simulink model "dft_8_point"  (R2016b)
settings: Solver=VariableStepDiscrete  StartTime=0.0  StopTime=12/fs  RelTol=1e-3  EnableMultiTasking=on
PreLoadFcn:
  | t = 2;
  | b = 14;
  | 
  | fs = 1;
StartFcn:
  | close all;
StopFcn:
  | % create matrices of Re and Im parts over time - inputs
  | xin_re = [xin_0_re xin_1_re xin_2_re xin_3_re xin_4_re xin_5_re xin_6_re xin_7_re];
  | xin_im = [xin_0_im xin_0_im xin_0_im xin_0_im xin_0_im xin_0_im xin_0_im xin_0_im];
  | 
  | % create matrices of Re and Im parts over time - outputs
  | X_re = [X0_re X1_re X2_re X3_re X4_re X5_re X6_re X7_re];
  | X_im = [X0_im X1_im X2_im X3_im X4_im X5_im X6_im X7_im];
  | 
  | % create vectors of Magnitudes and Angles over time
  | X_mag = [X0_mag X1_mag X2_mag X3_mag X4_mag X5_mag X6_mag X7_mag];
  | X_ang = [X0_ang X1_ang X2_ang X3_ang X4_ang X5_ang X6_ang X7_ang];
  | 
  | 
  | figure(1)
  | hold off
  | plot([0:1:7],xin_re(end,:),'r-o','MarkerFaceColor','r');
  | hold on
  | plot([0:1:7],xin_im(end,:),'b-o','MarkerFaceColor','b');
  | xlabel('Samples');
  | ylabel('Magnitude');
  | title('Input to DFT');
  | legend('Real','Imaginary','Location','EastOutside')
  | grid on;
  | 
  | set(1,'Name','Input to DFT','NumberTitle','off');
  | % setStandardFigSize(1);
  | 
  | figure(2)
  | hold off
  | plot([0:1:7],X_mag(end,:),'k-o','MarkerFaceColor','b');
  | hold on
  | xlabel('Frequency Bin');
  | ylabel('Magnitude');
  | grid on;
  | title('Magnitude DFT Plot');
  | 
  | set(2,'Name','Output of DFT','NumberTitle','off');
  | % setStandardFigSize(2);
libraries: xbsIndex_r4 x955
(part 1 of 8)
settings Model: Creator=lcrockett  LastModifiedBy=Administrator
settings DataIOCC: LimitDataPoints=on  SaveFormat=Array  SignalLoggingSaveFormat=ModelDataLogs
settings OptimizationCC: ExpressionDepthLimit=2147483647  LifeSpan=inf
settings DebuggingCC: UnderspecifiedInitializationDetection=Classic  MergeDetectMultiDrivingBlocksExec=none  SolverPrmCheckMsg=warning  FcnCallInpInsideContextMsg=warning  StateNameClashWarn=warning  SFUnexpectedBacktrackingDiag=warning  SFNoUnconditionalDefaultTransitionDiag=warning  SFExecutionAtInitializationDiag=none
settings HardwareCC: ProdBitPerPointer=32  ProdBitPerSizeT=32  ProdBitPerPtrDiffT=32  ProdLargestAtomicFloat=None  ProdIntDivRoundTo=Undefined  ProdEndianess=Unspecified  ProdWordSize=32  ProdHWDeviceType=32-bit Generic
settings ModelReferenceCC: PropagateSignalLabelsOutOfModel=off
settings GRTTargetCC: TargetLangStandard=C89/C90 (ANSI)  GeneratePreprocessorConditionals=Disable all  CombineOutputUpdateFcns=off  GRTInterface=on
settings ConfigComp: CovMetricSettings=dw  CovHtmlReporting=on  CovSaveCumulativeToWorkspaceVar=on  CovSaveSingleToWorkspaceVar=on  CovExternalEMLEnable=off

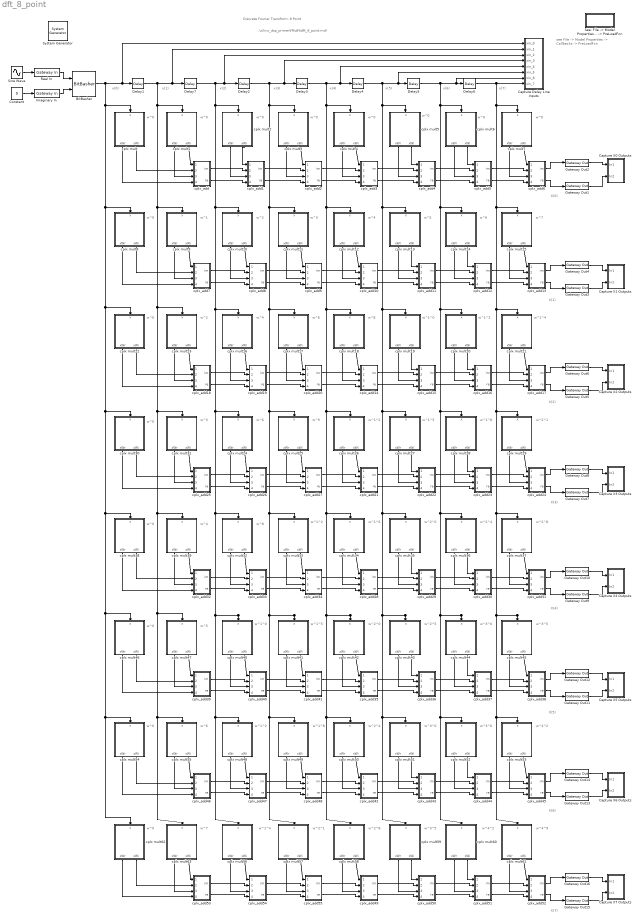
== system dft_8_point ==
  note: w^0
  note: w^0
  note: w^0
  note: w^0
  note: w^0
  note: w^0
  note: w^0
  note: w^0
  note: w^0
  note: w^0
  note: w^0
  note: w^0
  note: w^0
  note: w^0
  note: w^0
  note: w^1
  note: w^2
  note: w^2
  note: w^3
  note: w^3
  note: w^4
  note: w^4
  note: w^5
  note: w^6
  note: w^7
  note: w^5
  note: w^6
  note: w^7
  note: w^4
  note: w^6
  note: w^8
  note: w^1^0
  note: w^1^2
  note: w^1^4
  note: w^6
  note: w^9
  note: w^1^2
  note: w^1^5
  note: w^1^8
  note: w^2^1
  note: w^8
  note: w^1^2
  note: w^1^6
  note: w^2^0
  note: w^2^4
  note: w^2^8
  note: w^1^0
  note: w^1^5
  note: w^2^0
  note: w^2^5
  note: w^3^0
  note: w^3^5
  note: w^1^2
  note: w^1^8
  note: w^2^4
  note: w^3^0
  note: w^3^6
  note: w^4^2
  note: w^1^4
  note: w^2^1
  note: w^2^8
  note: w^3^5
  note: w^4^2
  note: w^4^9
  note: Discrete Fourier Transform: 8 Point
  note: ..\xilinx_dsp_primer\fft\dft\dft_8_point.mdl
  note: see File -> Model Properties
      | -> Callbacks -> PreLoadFcn
  note: x(0)
  note: x(1)
  note: x(2)
  note: x(3)
  note: x(4)
  note: x(5)
  note: x(6)
  note: x(7)
  note: X(0)
  note: X(1)
  note: X(2)
  note: X(3)
  note: X(4)
  note: X(5)
  note: X(6)
  note: X(7)
  " System Generator" : xbsIndex_r4/ System Generator  Tag=genX  xilinxfamily=artix7  part=xc7a75t  speed=-1  package=fgg484  synthesis_tool=Vivado  clock_wrapper=Clock Enables  directory=./netlist  proj_type=Vivado  Synth_file=Vivado Synthesis Defaults  Impl_file=Vivado Implementation Defaults  testbench=off  simulink_period=1/fs  sysclk_period=10  dcm_input_clock_period=10  incr_netlist=off  trim_vbits=Everywhere in SubSystem  dbl_ovrd=According to Block Masks  core_generation=According to Block Masks  run_coregen=off  deprecated_control=off  eval_field=0  block_type=sysgen
  BitBasher : xbsIndex_r4/BitBasher  bitexpr=|  display_expr=on  sr_1=1  arith_type1=Unsigned  bin_pt1=0  sr_2=2  arith_type2=Unsigned  bin_pt2=0  sr_3=3  arith_type3=Unsigned  bin_pt3=0  sr_4=4  arith_type4=Unsigned  bin_pt4=0  dbl_ovrd=off  block_type=bitbasher
      | <!DOCTYPE HTML PUBLIC "-//W3C//DTD HTML 4.0//EN" "http://www.w3.org/TR/REC-html40/strict.dtd">
      | <html><head><meta name="qrichtext" content="1" /><style type="text/css">
      | p, li { white-space: pre-wrap; }
      | </style></head><body style=" font-family:'MS Shell Dlg 2'; font-size:8.25pt; font-weight:400; font-style:normal;">
      | <p style=" margin-top:12px; margin-bottom:12px; margin-left:0px; margin-right:0px; -qt-block-indent:0; text-indent:0px;"><span style=" font-family:'MS Shell Dlg'; font-size:8pt;">a={b,c}</span></p></body></html>
  Capture X0 Outputs : Subsystem
  Capture X2 Outputs : Subsystem
  Capture X6 Outputs : Subsystem
  Capture X1 Outputs : Subsystem
  Capture X3 Outputs : Subsystem
  Capture X4 Outputs : Subsystem
  Capture X5 Outputs : Subsystem
  Capture X7 Outputs : Subsystem
  Capture Delay Line Inputs : Subsystem
  Constant : Constant  Value=0
  Delay{1..7} (7 alike) : xbsIndex_r4/Delay  rst=off  infoeditControl=Selection of Reset will increase slice count due to use of real FFs and instead of SRLs  en=off  latency=1  reg_retiming=off  dbl_ovrd=off  block_type=delay
  Gateway Out{1..16} (16 alike) : xbsIndex_r4/Gateway Out  inherit_from_input=off  hdl_port=on  rows=1  columns=1  UseAsDAC=off  DACChannel='1'  interface=None  automatic_assignment=on  address_offset=hex2dec('00')  intf_name=''  intf_description=''  timing_constraint=None  locs_specified=off  LOCs={}  io_standard={}  block_type=gatewayout
      settings: infoedit="Gateway out block.  Converts Xilinx fixed point inputs into ouputs of type Simulink integer, double, or fixed point.<br><br>Hardware notes:  In hardware these blocks become top level output ports or are discarded, depending on how they are configured."
  Imaginary In : xbsIndex_r4/Gateway In  gui_display_data_type=Fixed-point  arith_type="Signed  (2's comp)"  n_bits=t+b  bin_pt=b  preci_type=Single  exp_width=8  frac_width=24  rows=1  columns=1  quantization="Round  (unbiased: +/- Inf)"  overflow=Saturate  period=1/fs  UseAsADC=off  ADCChannel='1'  interface=None  automatic_assignment=on  address_offset=hex2dec('00')  intf_name=''  intf_description=''  default_value=0  timing_constraint=None  locs_specified=off  LOCs={}  io_standard={}  inherit_from_input=off  hdl_port=on  dbl_ovrd=off  block_type=gatewayin
      settings: infoedit="Gateway in block.  Converts inputs of type Simulink integer, double and fixed point to  Xilinx fixed point type.<br><br>Hardware notes:  In hardware these blocks become top level input ports."
  Real In : xbsIndex_r4/Gateway In  gui_display_data_type=Fixed-point  arith_type="Signed  (2's comp)"  n_bits=t+b  bin_pt=b  preci_type=Single  exp_width=8  frac_width=24  rows=1  columns=1  quantization="Round  (unbiased: +/- Inf)"  overflow=Saturate  period=1/fs  UseAsADC=off  ADCChannel='1'  interface=None  automatic_assignment=on  address_offset=hex2dec('00')  intf_name=''  intf_description=''  default_value=0  timing_constraint=None  locs_specified=off  LOCs={}  io_standard={}  inherit_from_input=off  hdl_port=on  dbl_ovrd=off  block_type=gatewayin
      settings: infoedit="Gateway in block.  Converts inputs of type Simulink integer, double and fixed point to  Xilinx fixed point type.<br><br>Hardware notes:  In hardware these blocks become top level input ports."
  "See: File -> Model Properties -> Callbacks -> PreLoadFcn " : Subsystem
      mask Display:
      | MHz = evalin('base', 'MHz');
      | fprintf(['fs = ',num2str(MHz),' MHz']);
  Sine Wave : Sin  Frequency=fs*2*pi/8  SampleTime=0
  cplx mult : Subsystem  mask(Complex Multiplier for DFT){n=0, k=0}
      mask prompts: n "Signal sample index, n"; k "Frequency index, k"
      mask help: This subsystem will multiply a complex input signal, x, with a complex weight value for the DFT/FFT, as defined via the mask.
      mask init:
      | t = evalin('base','t');   % integer bits
      | b = evalin('base','b');   % fractional bits   
      | N = 8;                    % size of FFT
      | W = exp(-1j*2*pi/N);      % the constant W
      | Wnk = W^(n*k);            % the complex twiddle factor for n,k
      | %W_nk_re = real(Wnk);
      | %W_nk_im = imag(Wnk);
      mask Display:
      | %plot([0.5 0.5+(real(Wnk)/0.5)],[0.5 0.5+(imag(Wnk)/0.5)]);
      | fprintf('Re = %+0.3f\r\nIm = %+0.3f',  real(Wnk), imag(Wnk));
  cplx mult1 : Subsystem  mask(Complex Multiplier for DFT){n=1, k=0}
      mask prompts: n "Signal sample index, n"; k "Frequency index, k"
      mask help: This subsystem will multiply a complex input signal, x, with a complex weight value for the DFT/FFT, as defined via the mask.
      mask init: same as dft_8_point/cplx mult
      mask Display:
      | %plot([0.5 0.5+(real(Wnk)/0.5)],[0.5 0.5+(imag(Wnk)/0.5)]);
      | fprintf('Re = %+0.3f\r\nIm = %+0.3f',  real(Wnk), imag(Wnk));
  cplx mult10 : Subsystem  mask(Complex Multiplier for DFT){n=2, k=1}
      mask prompts: n "Signal sample index, n"; k "Frequency index, k"
      mask help: This subsystem will multiply a complex input signal, x, with a complex weight value for the DFT/FFT, as defined via the mask.
      mask init: same as dft_8_point/cplx mult
      mask Display:
      | %plot([0.5 0.5+(real(Wnk)/0.5)],[0.5 0.5+(imag(Wnk)/0.5)]);
      | fprintf('Re = %+0.3f\r\nIm = %+0.3f',  real(Wnk), imag(Wnk));
  cplx mult11 : Subsystem  mask(Complex Multiplier for DFT){n=3, k=1}
      mask prompts: n "Signal sample index, n"; k "Frequency index, k"
      mask help: This subsystem will multiply a complex input signal, x, with a complex weight value for the DFT/FFT, as defined via the mask.
      mask init: same as dft_8_point/cplx mult
      mask Display:
      | %plot([0.5 0.5+(real(Wnk)/0.5)],[0.5 0.5+(imag(Wnk)/0.5)]);
      | fprintf('Re = %+0.3f\r\nIm = %+0.3f',  real(Wnk), imag(Wnk));
  cplx mult12 : Subsystem  mask(Complex Multiplier for DFT){n=4, k=1}
      mask prompts: n "Signal sample index, n"; k "Frequency index, k"
      mask help: This subsystem will multiply a complex input signal, x, with a complex weight value for the DFT/FFT, as defined via the mask.
      mask init: same as dft_8_point/cplx mult
      mask Display:
      | %plot([0.5 0.5+(real(Wnk)/0.5)],[0.5 0.5+(imag(Wnk)/0.5)]);
      | fprintf('Re = %+0.3f\r\nIm = %+0.3f',  real(Wnk), imag(Wnk));
  cplx mult13 : Subsystem  mask(Complex Multiplier for DFT){n=5, k=1}
      mask prompts: n "Signal sample index, n"; k "Frequency index, k"
      mask help: This subsystem will multiply a complex input signal, x, with a complex weight value for the DFT/FFT, as defined via the mask.
      mask init: same as dft_8_point/cplx mult
      mask Display:
      | %plot([0.5 0.5+(real(Wnk)/0.5)],[0.5 0.5+(imag(Wnk)/0.5)]);
      | fprintf('Re = %+0.3f\r\nIm = %+0.3f',  real(Wnk), imag(Wnk));
  cplx mult14 : Subsystem  mask(Complex Multiplier for DFT){n=6, k=1}
      mask prompts: n "Signal sample index, n"; k "Frequency index, k"
      mask help: This subsystem will multiply a complex input signal, x, with a complex weight value for the DFT/FFT, as defined via the mask.
      mask init: same as dft_8_point/cplx mult
      mask Display:
      | %plot([0.5 0.5+(real(Wnk)/0.5)],[0.5 0.5+(imag(Wnk)/0.5)]);
      | fprintf('Re = %+0.3f\r\nIm = %+0.3f',  real(Wnk), imag(Wnk));
  cplx mult15 : Subsystem  mask(Complex Multiplier for DFT){n=7, k=1}
      mask prompts: n "Signal sample index, n"; k "Frequency index, k"
      mask help: This subsystem will multiply a complex input signal, x, with a complex weight value for the DFT/FFT, as defined via the mask.
      mask init: same as dft_8_point/cplx mult
      mask Display:
      | %plot([0.5 0.5+(real(Wnk)/0.5)],[0.5 0.5+(imag(Wnk)/0.5)]);
      | fprintf('Re = %+0.3f\r\nIm = %+0.3f',  real(Wnk), imag(Wnk));
  cplx mult16 : Subsystem  mask(Complex Multiplier for DFT){n=2, k=2}
      mask prompts: n "Signal sample index, n"; k "Frequency index, k"
      mask help: This subsystem will multiply a complex input signal, x, with a complex weight value for the DFT/FFT, as defined via the mask.
      mask init: same as dft_8_point/cplx mult
      mask Display:
      | %plot([0.5 0.5+(real(Wnk)/0.5)],[0.5 0.5+(imag(Wnk)/0.5)]);
      | fprintf('Re = %+0.3f\r\nIm = %+0.3f',  real(Wnk), imag(Wnk));
  cplx mult17 : Subsystem  mask(Complex Multiplier for DFT){n=3, k=2}
      mask prompts: n "Signal sample index, n"; k "Frequency index, k"
      mask help: This subsystem will multiply a complex input signal, x, with a complex weight value for the DFT/FFT, as defined via the mask.
      mask init: same as dft_8_point/cplx mult
      mask Display:
      | %plot([0.5 0.5+(real(Wnk)/0.5)],[0.5 0.5+(imag(Wnk)/0.5)]);
      | fprintf('Re = %+0.3f\r\nIm = %+0.3f',  real(Wnk), imag(Wnk));
  cplx mult18 : Subsystem  mask(Complex Multiplier for DFT){n=4, k=2}
      mask prompts: n "Signal sample index, n"; k "Frequency index, k"
      mask help: This subsystem will multiply a complex input signal, x, with a complex weight value for the DFT/FFT, as defined via the mask.
      mask init: same as dft_8_point/cplx mult
      mask Display:
      | %plot([0.5 0.5+(real(Wnk)/0.5)],[0.5 0.5+(imag(Wnk)/0.5)]);
      | fprintf('Re = %+0.3f\r\nIm = %+0.3f',  real(Wnk), imag(Wnk));
  cplx mult19 : Subsystem  mask(Complex Multiplier for DFT){n=5, k=2}
      mask prompts: n "Signal sample index, n"; k "Frequency index, k"
      mask help: This subsystem will multiply a complex input signal, x, with a complex weight value for the DFT/FFT, as defined via the mask.
      mask init: same as dft_8_point/cplx mult
      mask Display:
      | %plot([0.5 0.5+(real(Wnk)/0.5)],[0.5 0.5+(imag(Wnk)/0.5)]);
      | fprintf('Re = %+0.3f\r\nIm = %+0.3f',  real(Wnk), imag(Wnk));
  cplx mult2 : Subsystem  mask(Complex Multiplier for DFT){n=2, k=0}
      mask prompts: n "Signal sample index, n"; k "Frequency index, k"
      mask help: This subsystem will multiply a complex input signal, x, with a complex weight value for the DFT/FFT, as defined via the mask.
      mask init: same as dft_8_point/cplx mult
      mask Display:
      | %plot([0.5 0.5+(real(Wnk)/0.5)],[0.5 0.5+(imag(Wnk)/0.5)]);
      | fprintf('Re = %+0.3f\r\nIm = %+0.3f',  real(Wnk), imag(Wnk));
  cplx mult20 : Subsystem  mask(Complex Multiplier for DFT){n=6, k=2}
      mask prompts: n "Signal sample index, n"; k "Frequency index, k"
      mask help: This subsystem will multiply a complex input signal, x, with a complex weight value for the DFT/FFT, as defined via the mask.
      mask init: same as dft_8_point/cplx mult
      mask Display:
      | %plot([0.5 0.5+(real(Wnk)/0.5)],[0.5 0.5+(imag(Wnk)/0.5)]);
      | fprintf('Re = %+0.3f\r\nIm = %+0.3f',  real(Wnk), imag(Wnk));
  cplx mult21 : Subsystem  mask(Complex Multiplier for DFT){n=7, k=2}
      mask prompts: n "Signal sample index, n"; k "Frequency index, k"
      mask help: This subsystem will multiply a complex input signal, x, with a complex weight value for the DFT/FFT, as defined via the mask.
      mask init: same as dft_8_point/cplx mult
      mask Display:
      | %plot([0.5 0.5+(real(Wnk)/0.5)],[0.5 0.5+(imag(Wnk)/0.5)]);
      | fprintf('Re = %+0.3f\r\nIm = %+0.3f',  real(Wnk), imag(Wnk));
  cplx mult22 : Subsystem  mask(Complex Multiplier for DFT){n=0, k=2}
      mask prompts: n "Signal sample index, n"; k "Frequency index, k"
      mask help: This subsystem will multiply a complex input signal, x, with a complex weight value for the DFT/FFT, as defined via the mask.
      mask init: same as dft_8_point/cplx mult
      mask Display:
      | %plot([0.5 0.5+(real(Wnk)/0.5)],[0.5 0.5+(imag(Wnk)/0.5)]);
      | fprintf('Re = %+0.3f\r\nIm = %+0.3f',  real(Wnk), imag(Wnk));
  cplx mult23 : Subsystem  mask(Complex Multiplier for DFT){n=1, k=2}
      mask prompts: n "Signal sample index, n"; k "Frequency index, k"
      mask help: This subsystem will multiply a complex input signal, x, with a complex weight value for the DFT/FFT, as defined via the mask.
      mask init: same as dft_8_point/cplx mult
      mask Display:
      | %plot([0.5 0.5+(real(Wnk)/0.5)],[0.5 0.5+(imag(Wnk)/0.5)]);
      | fprintf('Re = %+0.3f\r\nIm = %+0.3f',  real(Wnk), imag(Wnk));
  cplx mult24 : Subsystem  mask(Complex Multiplier for DFT){n=2, k=3}
      mask prompts: n "Signal sample index, n"; k "Frequency index, k"
      mask help: This subsystem will multiply a complex input signal, x, with a complex weight value for the DFT/FFT, as defined via the mask.
      mask init: same as dft_8_point/cplx mult
      mask Display:
      | %plot([0.5 0.5+(real(Wnk)/0.5)],[0.5 0.5+(imag(Wnk)/0.5)]);
      | fprintf('Re = %+0.3f\r\nIm = %+0.3f',  real(Wnk), imag(Wnk));
  cplx mult25 : Subsystem  mask(Complex Multiplier for DFT){n=3, k=3}
      mask prompts: n "Signal sample index, n"; k "Frequency index, k"
      mask help: This subsystem will multiply a complex input signal, x, with a complex weight value for the DFT/FFT, as defined via the mask.
      mask init: same as dft_8_point/cplx mult
      mask Display:
      | %plot([0.5 0.5+(real(Wnk)/0.5)],[0.5 0.5+(imag(Wnk)/0.5)]);
      | fprintf('Re = %+0.3f\r\nIm = %+0.3f',  real(Wnk), imag(Wnk));
  cplx mult26 : Subsystem  mask(Complex Multiplier for DFT){n=4, k=3}
      mask prompts: n "Signal sample index, n"; k "Frequency index, k"
      mask help: This subsystem will multiply a complex input signal, x, with a complex weight value for the DFT/FFT, as defined via the mask.
      mask init: same as dft_8_point/cplx mult
      mask Display:
      | %plot([0.5 0.5+(real(Wnk)/0.5)],[0.5 0.5+(imag(Wnk)/0.5)]);
      | fprintf('Re = %+0.3f\r\nIm = %+0.3f',  real(Wnk), imag(Wnk));
  cplx mult27 : Subsystem  mask(Complex Multiplier for DFT){n=5, k=3}
      mask prompts: n "Signal sample index, n"; k "Frequency index, k"
      mask help: This subsystem will multiply a complex input signal, x, with a complex weight value for the DFT/FFT, as defined via the mask.
      mask init: same as dft_8_point/cplx mult
      mask Display:
      | %plot([0.5 0.5+(real(Wnk)/0.5)],[0.5 0.5+(imag(Wnk)/0.5)]);
      | fprintf('Re = %+0.3f\r\nIm = %+0.3f',  real(Wnk), imag(Wnk));
  cplx mult28 : Subsystem  mask(Complex Multiplier for DFT){n=6, k=3}
      mask prompts: n "Signal sample index, n"; k "Frequency index, k"
      mask help: This subsystem will multiply a complex input signal, x, with a complex weight value for the DFT/FFT, as defined via the mask.
      mask init: same as dft_8_point/cplx mult
      mask Display:
      | %plot([0.5 0.5+(real(Wnk)/0.5)],[0.5 0.5+(imag(Wnk)/0.5)]);
      | fprintf('Re = %+0.3f\r\nIm = %+0.3f',  real(Wnk), imag(Wnk));
  cplx mult29 : Subsystem  mask(Complex Multiplier for DFT){n=7, k=3}
      mask prompts: n "Signal sample index, n"; k "Frequency index, k"
      mask help: This subsystem will multiply a complex input signal, x, with a complex weight value for the DFT/FFT, as defined via the mask.
      mask init: same as dft_8_point/cplx mult
      mask Display:
      | %plot([0.5 0.5+(real(Wnk)/0.5)],[0.5 0.5+(imag(Wnk)/0.5)]);
      | fprintf('Re = %+0.3f\r\nIm = %+0.3f',  real(Wnk), imag(Wnk));
  cplx mult3 : Subsystem  mask(Complex Multiplier for DFT){n=3, k=0}
      mask prompts: n "Signal sample index, n"; k "Frequency index, k"
      mask help: This subsystem will multiply a complex input signal, x, with a complex weight value for the DFT/FFT, as defined via the mask.
      mask init: same as dft_8_point/cplx mult
      mask Display:
      | %plot([0.5 0.5+(real(Wnk)/0.5)],[0.5 0.5+(imag(Wnk)/0.5)]);
      | fprintf('Re = %+0.3f\r\nIm = %+0.3f',  real(Wnk), imag(Wnk));
  cplx mult30 : Subsystem  mask(Complex Multiplier for DFT){n=0, k=3}
      mask prompts: n "Signal sample index, n"; k "Frequency index, k"
      mask help: This subsystem will multiply a complex input signal, x, with a complex weight value for the DFT/FFT, as defined via the mask.
      mask init: same as dft_8_point/cplx mult
      mask Display:
      | %plot([0.5 0.5+(real(Wnk)/0.5)],[0.5 0.5+(imag(Wnk)/0.5)]);
      | fprintf('Re = %+0.3f\r\nIm = %+0.3f',  real(Wnk), imag(Wnk));
  cplx mult31 : Subsystem  mask(Complex Multiplier for DFT){n=1, k=3}
      mask prompts: n "Signal sample index, n"; k "Frequency index, k"
      mask help: This subsystem will multiply a complex input signal, x, with a complex weight value for the DFT/FFT, as defined via the mask.
      mask init: same as dft_8_point/cplx mult
      mask Display:
      | %plot([0.5 0.5+(real(Wnk)/0.5)],[0.5 0.5+(imag(Wnk)/0.5)]);
      | fprintf('Re = %+0.3f\r\nIm = %+0.3f',  real(Wnk), imag(Wnk));
  cplx mult32 : Subsystem  mask(Complex Multiplier for DFT){n=2, k=4}
      mask prompts: n "Signal sample index, n"; k "Frequency index, k"
      mask help: This subsystem will multiply a complex input signal, x, with a complex weight value for the DFT/FFT, as defined via the mask.
      mask init: same as dft_8_point/cplx mult
      mask Display:
      | %plot([0.5 0.5+(real(Wnk)/0.5)],[0.5 0.5+(imag(Wnk)/0.5)]);
      | fprintf('Re = %+0.3f\r\nIm = %+0.3f',  real(Wnk), imag(Wnk));
  cplx mult33 : Subsystem  mask(Complex Multiplier for DFT){n=3, k=4}
      mask prompts: n "Signal sample index, n"; k "Frequency index, k"
      mask help: This subsystem will multiply a complex input signal, x, with a complex weight value for the DFT/FFT, as defined via the mask.
      mask init: same as dft_8_point/cplx mult
      mask Display:
      | %plot([0.5 0.5+(real(Wnk)/0.5)],[0.5 0.5+(imag(Wnk)/0.5)]);
      | fprintf('Re = %+0.3f\r\nIm = %+0.3f',  real(Wnk), imag(Wnk));
  cplx mult34 : Subsystem  mask(Complex Multiplier for DFT){n=4, k=4}
      mask prompts: n "Signal sample index, n"; k "Frequency index, k"
      mask help: This subsystem will multiply a complex input signal, x, with a complex weight value for the DFT/FFT, as defined via the mask.
      mask init: same as dft_8_point/cplx mult
      mask Display:
      | %plot([0.5 0.5+(real(Wnk)/0.5)],[0.5 0.5+(imag(Wnk)/0.5)]);
      | fprintf('Re = %+0.3f\r\nIm = %+0.3f',  real(Wnk), imag(Wnk));
  cplx mult35 : Subsystem  mask(Complex Multiplier for DFT){n=5, k=4}
      mask prompts: n "Signal sample index, n"; k "Frequency index, k"
      mask help: This subsystem will multiply a complex input signal, x, with a complex weight value for the DFT/FFT, as defined via the mask.
      mask init: same as dft_8_point/cplx mult
      mask Display:
      | %plot([0.5 0.5+(real(Wnk)/0.5)],[0.5 0.5+(imag(Wnk)/0.5)]);
      | fprintf('Re = %+0.3f\r\nIm = %+0.3f',  real(Wnk), imag(Wnk));
  cplx mult36 : Subsystem  mask(Complex Multiplier for DFT){n=6, k=4}
      mask prompts: n "Signal sample index, n"; k "Frequency index, k"
      mask help: This subsystem will multiply a complex input signal, x, with a complex weight value for the DFT/FFT, as defined via the mask.
      mask init: same as dft_8_point/cplx mult
      mask Display:
      | %plot([0.5 0.5+(real(Wnk)/0.5)],[0.5 0.5+(imag(Wnk)/0.5)]);
      | fprintf('Re = %+0.3f\r\nIm = %+0.3f',  real(Wnk), imag(Wnk));
  cplx mult37 : Subsystem  mask(Complex Multiplier for DFT){n=7, k=4}
      mask prompts: n "Signal sample index, n"; k "Frequency index, k"
      mask help: This subsystem will multiply a complex input signal, x, with a complex weight value for the DFT/FFT, as defined via the mask.
      mask init: same as dft_8_point/cplx mult
      mask Display:
      | %plot([0.5 0.5+(real(Wnk)/0.5)],[0.5 0.5+(imag(Wnk)/0.5)]);
      | fprintf('Re = %+0.3f\r\nIm = %+0.3f',  real(Wnk), imag(Wnk));
  cplx mult38 : Subsystem  mask(Complex Multiplier for DFT){n=0, k=4}
      mask prompts: n "Signal sample index, n"; k "Frequency index, k"
      mask help: This subsystem will multiply a complex input signal, x, with a complex weight value for the DFT/FFT, as defined via the mask.
      mask init: same as dft_8_point/cplx mult
      mask Display:
      | %plot([0.5 0.5+(real(Wnk)/0.5)],[0.5 0.5+(imag(Wnk)/0.5)]);
      | fprintf('Re = %+0.3f\r\nIm = %+0.3f',  real(Wnk), imag(Wnk));
  cplx mult39 : Subsystem  mask(Complex Multiplier for DFT){n=1, k=4}
      mask prompts: n "Signal sample index, n"; k "Frequency index, k"
      mask help: This subsystem will multiply a complex input signal, x, with a complex weight value for the DFT/FFT, as defined via the mask.
      mask init: same as dft_8_point/cplx mult
      mask Display:
      | %plot([0.5 0.5+(real(Wnk)/0.5)],[0.5 0.5+(imag(Wnk)/0.5)]);
      | fprintf('Re = %+0.3f\r\nIm = %+0.3f',  real(Wnk), imag(Wnk));
  cplx mult4 : Subsystem  mask(Complex Multiplier for DFT){n=4, k=0}
      mask prompts: n "Signal sample index, n"; k "Frequency index, k"
      mask help: This subsystem will multiply a complex input signal, x, with a complex weight value for the DFT/FFT, as defined via the mask.
      mask init: same as dft_8_point/cplx mult
      mask Display:
      | %plot([0.5 0.5+(real(Wnk)/0.5)],[0.5 0.5+(imag(Wnk)/0.5)]);
      | fprintf('Re = %+0.3f\r\nIm = %+0.3f',  real(Wnk), imag(Wnk));
  cplx mult40 : Subsystem  mask(Complex Multiplier for DFT){n=2, k=5}
      mask prompts: n "Signal sample index, n"; k "Frequency index, k"
      mask help: This subsystem will multiply a complex input signal, x, with a complex weight value for the DFT/FFT, as defined via the mask.
      mask init: same as dft_8_point/cplx mult
      mask Display:
      | %plot([0.5 0.5+(real(Wnk)/0.5)],[0.5 0.5+(imag(Wnk)/0.5)]);
      | fprintf('Re = %+0.3f\r\nIm = %+0.3f',  real(Wnk), imag(Wnk));
  cplx mult41 : Subsystem  mask(Complex Multiplier for DFT){n=3, k=5}
      mask prompts: n "Signal sample index, n"; k "Frequency index, k"
      mask help: This subsystem will multiply a complex input signal, x, with a complex weight value for the DFT/FFT, as defined via the mask.
      mask init: same as dft_8_point/cplx mult
      mask Display:
      | %plot([0.5 0.5+(real(Wnk)/0.5)],[0.5 0.5+(imag(Wnk)/0.5)]);
      | fprintf('Re = %+0.3f\r\nIm = %+0.3f',  real(Wnk), imag(Wnk));
  cplx mult42 : Subsystem  mask(Complex Multiplier for DFT){n=4, k=5}
      mask prompts: n "Signal sample index, n"; k "Frequency index, k"
      mask help: This subsystem will multiply a complex input signal, x, with a complex weight value for the DFT/FFT, as defined via the mask.
      mask init: same as dft_8_point/cplx mult
      mask Display:
      | %plot([0.5 0.5+(real(Wnk)/0.5)],[0.5 0.5+(imag(Wnk)/0.5)]);
      | fprintf('Re = %+0.3f\r\nIm = %+0.3f',  real(Wnk), imag(Wnk));
  cplx mult43 : Subsystem  mask(Complex Multiplier for DFT){n=5, k=5}
      mask prompts: n "Signal sample index, n"; k "Frequency index, k"
      mask help: This subsystem will multiply a complex input signal, x, with a complex weight value for the DFT/FFT, as defined via the mask.
      mask init: same as dft_8_point/cplx mult
      mask Display:
      | %plot([0.5 0.5+(real(Wnk)/0.5)],[0.5 0.5+(imag(Wnk)/0.5)]);
      | fprintf('Re = %+0.3f\r\nIm = %+0.3f',  real(Wnk), imag(Wnk));
  cplx mult44 : Subsystem  mask(Complex Multiplier for DFT){n=6, k=5}
      mask prompts: n "Signal sample index, n"; k "Frequency index, k"
      mask help: This subsystem will multiply a complex input signal, x, with a complex weight value for the DFT/FFT, as defined via the mask.
      mask init: same as dft_8_point/cplx mult
      mask Display:
      | %plot([0.5 0.5+(real(Wnk)/0.5)],[0.5 0.5+(imag(Wnk)/0.5)]);
      | fprintf('Re = %+0.3f\r\nIm = %+0.3f',  real(Wnk), imag(Wnk));
  cplx mult45 : Subsystem  mask(Complex Multiplier for DFT){n=7, k=5}
      mask prompts: n "Signal sample index, n"; k "Frequency index, k"
      mask help: This subsystem will multiply a complex input signal, x, with a complex weight value for the DFT/FFT, as defined via the mask.
      mask init: same as dft_8_point/cplx mult
      mask Display:
      | %plot([0.5 0.5+(real(Wnk)/0.5)],[0.5 0.5+(imag(Wnk)/0.5)]);
      | fprintf('Re = %+0.3f\r\nIm = %+0.3f',  real(Wnk), imag(Wnk));
  cplx mult46 : Subsystem  mask(Complex Multiplier for DFT){n=0, k=5}
      mask prompts: n "Signal sample index, n"; k "Frequency index, k"
      mask help: This subsystem will multiply a complex input signal, x, with a complex weight value for the DFT/FFT, as defined via the mask.
      mask init: same as dft_8_point/cplx mult
      mask Display:
      | %plot([0.5 0.5+(real(Wnk)/0.5)],[0.5 0.5+(imag(Wnk)/0.5)]);
      | fprintf('Re = %+0.3f\r\nIm = %+0.3f',  real(Wnk), imag(Wnk));
  cplx mult47 : Subsystem  mask(Complex Multiplier for DFT){n=1, k=5}
      mask prompts: n "Signal sample index, n"; k "Frequency index, k"
      mask help: This subsystem will multiply a complex input signal, x, with a complex weight value for the DFT/FFT, as defined via the mask.
      mask init: same as dft_8_point/cplx mult
      mask Display:
      | %plot([0.5 0.5+(real(Wnk)/0.5)],[0.5 0.5+(imag(Wnk)/0.5)]);
      | fprintf('Re = %+0.3f\r\nIm = %+0.3f',  real(Wnk), imag(Wnk));
  cplx mult48 : Subsystem  mask(Complex Multiplier for DFT){n=2, k=6}
      mask prompts: n "Signal sample index, n"; k "Frequency index, k"
      mask help: This subsystem will multiply a complex input signal, x, with a complex weight value for the DFT/FFT, as defined via the mask.
      mask init: same as dft_8_point/cplx mult
      mask Display:
      | %plot([0.5 0.5+(real(Wnk)/0.5)],[0.5 0.5+(imag(Wnk)/0.5)]);
      | fprintf('Re = %+0.3f\r\nIm = %+0.3f',  real(Wnk), imag(Wnk));
  cplx mult49 : Subsystem  mask(Complex Multiplier for DFT){n=3, k=6}
      mask prompts: n "Signal sample index, n"; k "Frequency index, k"
      mask help: This subsystem will multiply a complex input signal, x, with a complex weight value for the DFT/FFT, as defined via the mask.
      mask init: same as dft_8_point/cplx mult
      mask Display:
      | %plot([0.5 0.5+(real(Wnk)/0.5)],[0.5 0.5+(imag(Wnk)/0.5)]);
      | fprintf('Re = %+0.3f\r\nIm = %+0.3f',  real(Wnk), imag(Wnk));
  cplx mult5 : Subsystem  mask(Complex Multiplier for DFT){n=5, k=0}
      mask prompts: n "Signal sample index, n"; k "Frequency index, k"
      mask help: This subsystem will multiply a complex input signal, x, with a complex weight value for the DFT/FFT, as defined via the mask.
      mask init: same as dft_8_point/cplx mult
      mask Display:
      | %plot([0.5 0.5+(real(Wnk)/0.5)],[0.5 0.5+(imag(Wnk)/0.5)]);
      | fprintf('Re = %+0.3f\r\nIm = %+0.3f',  real(Wnk), imag(Wnk));
  cplx mult50 : Subsystem  mask(Complex Multiplier for DFT){n=4, k=6}
      mask prompts: n "Signal sample index, n"; k "Frequency index, k"
      mask help: This subsystem will multiply a complex input signal, x, with a complex weight value for the DFT/FFT, as defined via the mask.
      mask init: same as dft_8_point/cplx mult
      mask Display:
      | %plot([0.5 0.5+(real(Wnk)/0.5)],[0.5 0.5+(imag(Wnk)/0.5)]);
      | fprintf('Re = %+0.3f\r\nIm = %+0.3f',  real(Wnk), imag(Wnk));
  cplx mult51 : Subsystem  mask(Complex Multiplier for DFT){n=5, k=6}
      mask prompts: n "Signal sample index, n"; k "Frequency index, k"
      mask help: This subsystem will multiply a complex input signal, x, with a complex weight value for the DFT/FFT, as defined via the mask.
      mask init: same as dft_8_point/cplx mult
      mask Display:
      | %plot([0.5 0.5+(real(Wnk)/0.5)],[0.5 0.5+(imag(Wnk)/0.5)]);
      | fprintf('Re = %+0.3f\r\nIm = %+0.3f',  real(Wnk), imag(Wnk));
  cplx mult52 : Subsystem  mask(Complex Multiplier for DFT){n=6, k=6}
      mask prompts: n "Signal sample index, n"; k "Frequency index, k"
      mask help: This subsystem will multiply a complex input signal, x, with a complex weight value for the DFT/FFT, as defined via the mask.
      mask init: same as dft_8_point/cplx mult
      mask Display:
      | %plot([0.5 0.5+(real(Wnk)/0.5)],[0.5 0.5+(imag(Wnk)/0.5)]);
      | fprintf('Re = %+0.3f\r\nIm = %+0.3f',  real(Wnk), imag(Wnk));
  cplx mult53 : Subsystem  mask(Complex Multiplier for DFT){n=7, k=6}
      mask prompts: n "Signal sample index, n"; k "Frequency index, k"
      mask help: This subsystem will multiply a complex input signal, x, with a complex weight value for the DFT/FFT, as defined via the mask.
      mask init: same as dft_8_point/cplx mult
      mask Display:
      | %plot([0.5 0.5+(real(Wnk)/0.5)],[0.5 0.5+(imag(Wnk)/0.5)]);
      | fprintf('Re = %+0.3f\r\nIm = %+0.3f',  real(Wnk), imag(Wnk));
  cplx mult54 : Subsystem  mask(Complex Multiplier for DFT){n=0, k=6}
      mask prompts: n "Signal sample index, n"; k "Frequency index, k"
      mask help: This subsystem will multiply a complex input signal, x, with a complex weight value for the DFT/FFT, as defined via the mask.
      mask init: same as dft_8_point/cplx mult
      mask Display:
      | %plot([0.5 0.5+(real(Wnk)/0.5)],[0.5 0.5+(imag(Wnk)/0.5)]);
      | fprintf('Re = %+0.3f\r\nIm = %+0.3f',  real(Wnk), imag(Wnk));
  cplx mult55 : Subsystem  mask(Complex Multiplier for DFT){n=1, k=6}
      mask prompts: n "Signal sample index, n"; k "Frequency index, k"
      mask help: This subsystem will multiply a complex input signal, x, with a complex weight value for the DFT/FFT, as defined via the mask.
      mask init: same as dft_8_point/cplx mult
      mask Display:
      | %plot([0.5 0.5+(real(Wnk)/0.5)],[0.5 0.5+(imag(Wnk)/0.5)]);
      | fprintf('Re = %+0.3f\r\nIm = %+0.3f',  real(Wnk), imag(Wnk));
  cplx mult56 : Subsystem  mask(Complex Multiplier for DFT){n=2, k=7}
      mask prompts: n "Signal sample index, n"; k "Frequency index, k"
      mask help: This subsystem will multiply a complex input signal, x, with a complex weight value for the DFT/FFT, as defined via the mask.
      mask init: same as dft_8_point/cplx mult
      mask Display:
      | %plot([0.5 0.5+(real(Wnk)/0.5)],[0.5 0.5+(imag(Wnk)/0.5)]);
      | fprintf('Re = %+0.3f\r\nIm = %+0.3f',  real(Wnk), imag(Wnk));
  cplx mult57 : Subsystem  mask(Complex Multiplier for DFT){n=3, k=7}
      mask prompts: n "Signal sample index, n"; k "Frequency index, k"
      mask help: This subsystem will multiply a complex input signal, x, with a complex weight value for the DFT/FFT, as defined via the mask.
      mask init: same as dft_8_point/cplx mult
      mask Display:
      | %plot([0.5 0.5+(real(Wnk)/0.5)],[0.5 0.5+(imag(Wnk)/0.5)]);
      | fprintf('Re = %+0.3f\r\nIm = %+0.3f',  real(Wnk), imag(Wnk));
  cplx mult58 : Subsystem  mask(Complex Multiplier for DFT){n=4, k=7}
      mask prompts: n "Signal sample index, n"; k "Frequency index, k"
      mask help: This subsystem will multiply a complex input signal, x, with a complex weight value for the DFT/FFT, as defined via the mask.
      mask init: same as dft_8_point/cplx mult
      mask Display:
      | %plot([0.5 0.5+(real(Wnk)/0.5)],[0.5 0.5+(imag(Wnk)/0.5)]);
      | fprintf('Re = %+0.3f\r\nIm = %+0.3f',  real(Wnk), imag(Wnk));
  cplx mult59 : Subsystem  mask(Complex Multiplier for DFT){n=5, k=7}
      mask prompts: n "Signal sample index, n"; k "Frequency index, k"
      mask help: This subsystem will multiply a complex input signal, x, with a complex weight value for the DFT/FFT, as defined via the mask.
      mask init: same as dft_8_point/cplx mult
      mask Display:
      | %plot([0.5 0.5+(real(Wnk)/0.5)],[0.5 0.5+(imag(Wnk)/0.5)]);
      | fprintf('Re = %+0.3f\r\nIm = %+0.3f',  real(Wnk), imag(Wnk));
  cplx mult6 : Subsystem  mask(Complex Multiplier for DFT){n=6, k=0}
      mask prompts: n "Signal sample index, n"; k "Frequency index, k"
      mask help: This subsystem will multiply a complex input signal, x, with a complex weight value for the DFT/FFT, as defined via the mask.
      mask init: same as dft_8_point/cplx mult
      mask Display:
      | %plot([0.5 0.5+(real(Wnk)/0.5)],[0.5 0.5+(imag(Wnk)/0.5)]);
      | fprintf('Re = %+0.3f\r\nIm = %+0.3f',  real(Wnk), imag(Wnk));
  cplx mult60 : Subsystem  mask(Complex Multiplier for DFT){n=6, k=7}
      mask prompts: n "Signal sample index, n"; k "Frequency index, k"
      mask help: This subsystem will multiply a complex input signal, x, with a complex weight value for the DFT/FFT, as defined via the mask.
      mask init: same as dft_8_point/cplx mult
      mask Display:
      | %plot([0.5 0.5+(real(Wnk)/0.5)],[0.5 0.5+(imag(Wnk)/0.5)]);
      | fprintf('Re = %+0.3f\r\nIm = %+0.3f',  real(Wnk), imag(Wnk));
  cplx mult61 : Subsystem  mask(Complex Multiplier for DFT){n=7, k=7}
      mask prompts: n "Signal sample index, n"; k "Frequency index, k"
      mask help: This subsystem will multiply a complex input signal, x, with a complex weight value for the DFT/FFT, as defined via the mask.
      mask init: same as dft_8_point/cplx mult
      mask Display:
      | %plot([0.5 0.5+(real(Wnk)/0.5)],[0.5 0.5+(imag(Wnk)/0.5)]);
      | fprintf('Re = %+0.3f\r\nIm = %+0.3f',  real(Wnk), imag(Wnk));
  cplx mult62 : Subsystem  mask(Complex Multiplier for DFT){n=0, k=7}
      mask prompts: n "Signal sample index, n"; k "Frequency index, k"
      mask help: This subsystem will multiply a complex input signal, x, with a complex weight value for the DFT/FFT, as defined via the mask.
      mask init: same as dft_8_point/cplx mult
      mask Display:
      | %plot([0.5 0.5+(real(Wnk)/0.5)],[0.5 0.5+(imag(Wnk)/0.5)]);
      | fprintf('Re = %+0.3f\r\nIm = %+0.3f',  real(Wnk), imag(Wnk));
  cplx mult63 : Subsystem  mask(Complex Multiplier for DFT){n=1, k=7}
      mask prompts: n "Signal sample index, n"; k "Frequency index, k"
      mask help: This subsystem will multiply a complex input signal, x, with a complex weight value for the DFT/FFT, as defined via the mask.
      mask init: same as dft_8_point/cplx mult
      mask Display:
      | %plot([0.5 0.5+(real(Wnk)/0.5)],[0.5 0.5+(imag(Wnk)/0.5)]);
      | fprintf('Re = %+0.3f\r\nIm = %+0.3f',  real(Wnk), imag(Wnk));
  cplx mult7 : Subsystem  mask(Complex Multiplier for DFT){n=7, k=0}
      mask prompts: n "Signal sample index, n"; k "Frequency index, k"
      mask help: This subsystem will multiply a complex input signal, x, with a complex weight value for the DFT/FFT, as defined via the mask.
      mask init: same as dft_8_point/cplx mult
      mask Display:
      | %plot([0.5 0.5+(real(Wnk)/0.5)],[0.5 0.5+(imag(Wnk)/0.5)]);
      | fprintf('Re = %+0.3f\r\nIm = %+0.3f',  real(Wnk), imag(Wnk));
  cplx mult8 : Subsystem  mask(Complex Multiplier for DFT){n=0, k=1}
      mask prompts: n "Signal sample index, n"; k "Frequency index, k"
      mask help: This subsystem will multiply a complex input signal, x, with a complex weight value for the DFT/FFT, as defined via the mask.
      mask init: same as dft_8_point/cplx mult
      mask Display:
      | %plot([0.5 0.5+(real(Wnk)/0.5)],[0.5 0.5+(imag(Wnk)/0.5)]);
      | fprintf('Re = %+0.3f\r\nIm = %+0.3f',  real(Wnk), imag(Wnk));
  cplx mult9 : Subsystem  mask(Complex Multiplier for DFT){n=1, k=1}
      mask prompts: n "Signal sample index, n"; k "Frequency index, k"
      mask help: This subsystem will multiply a complex input signal, x, with a complex weight value for the DFT/FFT, as defined via the mask.
      mask init: same as dft_8_point/cplx mult
      mask Display:
      | %plot([0.5 0.5+(real(Wnk)/0.5)],[0.5 0.5+(imag(Wnk)/0.5)]);
      | fprintf('Re = %+0.3f\r\nIm = %+0.3f',  real(Wnk), imag(Wnk));
  cplx_add : Subsystem  mask(Complex Adder){t=t+2, b=b}
      mask prompts: t "Integer bits"; b "Fractional bits"
  cplx_add1 : Subsystem  mask(Complex Adder){t=t+3, b=b}
      mask prompts: t "Integer bits"; b "Fractional bits"
  cplx_add10 : Subsystem  mask(Complex Adder){t=t+4, b=b}
      mask prompts: t "Integer bits"; b "Fractional bits"
  cplx_add11 : Subsystem  mask(Complex Adder){t=t+4, b=b}
      mask prompts: t "Integer bits"; b "Fractional bits"
  cplx_add12 : Subsystem  mask(Complex Adder){t=t+4, b=b}
      mask prompts: t "Integer bits"; b "Fractional bits"
  cplx_add13 : Subsystem  mask(Complex Adder){t=t+4, b=b}
      mask prompts: t "Integer bits"; b "Fractional bits"
  cplx_add14 : Subsystem  mask(Complex Adder){t=t+4, b=b}
      mask prompts: t "Integer bits"; b "Fractional bits"
  cplx_add15 : Subsystem  mask(Complex Adder){t=t+4, b=b}
      mask prompts: t "Integer bits"; b "Fractional bits"
  cplx_add16 : Subsystem  mask(Complex Adder){t=t+4, b=b}
      mask prompts: t "Integer bits"; b "Fractional bits"
  cplx_add17 : Subsystem  mask(Complex Adder){t=t+4, b=b}
      mask prompts: t "Integer bits"; b "Fractional bits"
  cplx_add18 : Subsystem  mask(Complex Adder){t=t+2, b=b}
      mask prompts: t "Integer bits"; b "Fractional bits"
  cplx_add19 : Subsystem  mask(Complex Adder){t=t+3, b=b}
      mask prompts: t "Integer bits"; b "Fractional bits"
  cplx_add2 : Subsystem  mask(Complex Adder){t=t+3, b=b}
      mask prompts: t "Integer bits"; b "Fractional bits"
  cplx_add20 : Subsystem  mask(Complex Adder){t=t+3, b=b}
      mask prompts: t "Integer bits"; b "Fractional bits"
  cplx_add21 : Subsystem  mask(Complex Adder){t=t+4, b=b}
      mask prompts: t "Integer bits"; b "Fractional bits"
  cplx_add22 : Subsystem  mask(Complex Adder){t=t+4, b=b}
      mask prompts: t "Integer bits"; b "Fractional bits"
  cplx_add23 : Subsystem  mask(Complex Adder){t=t+4, b=b}
      mask prompts: t "Integer bits"; b "Fractional bits"
  cplx_add24 : Subsystem  mask(Complex Adder){t=t+4, b=b}
      mask prompts: t "Integer bits"; b "Fractional bits"
  cplx_add25 : Subsystem  mask(Complex Adder){t=t+2, b=b}
      mask prompts: t "Integer bits"; b "Fractional bits"
  cplx_add26 : Subsystem  mask(Complex Adder){t=t+3, b=b}
      mask prompts: t "Integer bits"; b "Fractional bits"
  cplx_add27 : Subsystem  mask(Complex Adder){t=t+3, b=b}
      mask prompts: t "Integer bits"; b "Fractional bits"
  cplx_add28 : Subsystem  mask(Complex Adder){t=t+4, b=b}
      mask prompts: t "Integer bits"; b "Fractional bits"
  cplx_add29 : Subsystem  mask(Complex Adder){t=t+4, b=b}
      mask prompts: t "Integer bits"; b "Fractional bits"
  cplx_add3 : Subsystem  mask(Complex Adder){t=t+4, b=b}
      mask prompts: t "Integer bits"; b "Fractional bits"
  cplx_add30 : Subsystem  mask(Complex Adder){t=t+4, b=b}
      mask prompts: t "Integer bits"; b "Fractional bits"
  cplx_add31 : Subsystem  mask(Complex Adder){t=t+4, b=b}
      mask prompts: t "Integer bits"; b "Fractional bits"
  cplx_add32 : Subsystem  mask(Complex Adder){t=t+2, b=b}
      mask prompts: t "Integer bits"; b "Fractional bits"
  cplx_add33 : Subsystem  mask(Complex Adder){t=t+3, b=b}
      mask prompts: t "Integer bits"; b "Fractional bits"
  cplx_add34 : Subsystem  mask(Complex Adder){t=t+3, b=b}
      mask prompts: t "Integer bits"; b "Fractional bits"
  cplx_add35 : Subsystem  mask(Complex Adder){t=t+4, b=b}
      mask prompts: t "Integer bits"; b "Fractional bits"
  cplx_add36 : Subsystem  mask(Complex Adder){t=t+4, b=b}
      mask prompts: t "Integer bits"; b "Fractional bits"
  cplx_add37 : Subsystem  mask(Complex Adder){t=t+4, b=b}
      mask prompts: t "Integer bits"; b "Fractional bits"
  cplx_add38 : Subsystem  mask(Complex Adder){t=t+4, b=b}
      mask prompts: t "Integer bits"; b "Fractional bits"
  cplx_add39 : Subsystem  mask(Complex Adder){t=t+2, b=b}
      mask prompts: t "Integer bits"; b "Fractional bits"
  cplx_add4 : Subsystem  mask(Complex Adder){t=t+4, b=b}
      mask prompts: t "Integer bits"; b "Fractional bits"
  cplx_add40 : Subsystem  mask(Complex Adder){t=t+3, b=b}
      mask prompts: t "Integer bits"; b "Fractional bits"
  cplx_add41 : Subsystem  mask(Complex Adder){t=t+3, b=b}
      mask prompts: t "Integer bits"; b "Fractional bits"
  cplx_add42 : Subsystem  mask(Complex Adder){t=t+4, b=b}
      mask prompts: t "Integer bits"; b "Fractional bits"
  cplx_add43 : Subsystem  mask(Complex Adder){t=t+4, b=b}
      mask prompts: t "Integer bits"; b "Fractional bits"
  cplx_add44 : Subsystem  mask(Complex Adder){t=t+4, b=b}
      mask prompts: t "Integer bits"; b "Fractional bits"
  cplx_add45 : Subsystem  mask(Complex Adder){t=t+4, b=b}
      mask prompts: t "Integer bits"; b "Fractional bits"
  cplx_add46 : Subsystem  mask(Complex Adder){t=t+2, b=b}
      mask prompts: t "Integer bits"; b "Fractional bits"
  cplx_add47 : Subsystem  mask(Complex Adder){t=t+3, b=b}
      mask prompts: t "Integer bits"; b "Fractional bits"
  cplx_add48 : Subsystem  mask(Complex Adder){t=t+3, b=b}
      mask prompts: t "Integer bits"; b "Fractional bits"
  cplx_add49 : Subsystem  mask(Complex Adder){t=t+4, b=b}
      mask prompts: t "Integer bits"; b "Fractional bits"
  cplx_add5 : Subsystem  mask(Complex Adder){t=t+4, b=b}
      mask prompts: t "Integer bits"; b "Fractional bits"
  cplx_add50 : Subsystem  mask(Complex Adder){t=t+4, b=b}
      mask prompts: t "Integer bits"; b "Fractional bits"
  cplx_add51 : Subsystem  mask(Complex Adder){t=t+4, b=b}
      mask prompts: t "Integer bits"; b "Fractional bits"
  cplx_add52 : Subsystem  mask(Complex Adder){t=t+4, b=b}
      mask prompts: t "Integer bits"; b "Fractional bits"
  cplx_add53 : Subsystem  mask(Complex Adder){t=t+2, b=b}
      mask prompts: t "Integer bits"; b "Fractional bits"
  cplx_add54 : Subsystem  mask(Complex Adder){t=t+3, b=b}
      mask prompts: t "Integer bits"; b "Fractional bits"
  cplx_add55 : Subsystem  mask(Complex Adder){t=t+3, b=b}
      mask prompts: t "Integer bits"; b "Fractional bits"
  cplx_add6 : Subsystem  mask(Complex Adder){t=t+4, b=b}
      mask prompts: t "Integer bits"; b "Fractional bits"
  cplx_add7 : Subsystem  mask(Complex Adder){t=t+2, b=b}
      mask prompts: t "Integer bits"; b "Fractional bits"
  cplx_add8 : Subsystem  mask(Complex Adder){t=t+3, b=b}
      mask prompts: t "Integer bits"; b "Fractional bits"
  cplx_add9 : Subsystem  mask(Complex Adder){t=t+3, b=b}
      mask prompts: t "Integer bits"; b "Fractional bits"
  wires:
  Delay2/1 -> cplx mult3/1(x), cplx mult11/1(x), cplx mult17/1(x), cplx mult25/1(x), cplx mult41/1(x), cplx mult49/1(x), cplx mult57/1(x), cplx mult33/1(x), Delay3/1, Capture Delay Line Inputs/4(xin_3)
  Delay3/1 -> cplx mult4/1(x), cplx mult12/1(x), cplx mult18/1(x), cplx mult26/1(x), cplx mult42/1(x), cplx mult50/1(x), cplx mult58/1(x), cplx mult34/1(x), Delay4/1, Capture Delay Line Inputs/5(xin_4)
  Delay4/1 -> cplx mult5/1(x), cplx mult13/1(x), cplx mult19/1(x), cplx mult27/1(x), cplx mult43/1(x), cplx mult51/1(x), cplx mult59/1(x), cplx mult35/1(x), Delay5/1, Capture Delay Line Inputs/6(xin_5)
  Delay5/1 -> cplx mult6/1(x), cplx mult14/1(x), cplx mult20/1(x), cplx mult28/1(x), cplx mult44/1(x), cplx mult52/1(x), cplx mult60/1(x), cplx mult36/1(x), Delay6/1, Capture Delay Line Inputs/7(xin_6)
  BitBasher/1 -> cplx mult8/1(x), cplx mult22/1(x), cplx mult30/1(x), cplx mult38/1(x), cplx mult46/1(x), cplx mult54/1(x), cplx mult62/1(x), cplx mult/1(x), Delay1/1, Capture Delay Line Inputs/1(xin_0)
  Delay6/1 -> cplx mult7/1(x), cplx mult15/1(x), cplx mult21/1(x), cplx mult29/1(x), cplx mult45/1(x), cplx mult53/1(x), cplx mult61/1(x), cplx mult37/1(x), Capture Delay Line Inputs/8(xin_7)
  Imaginary In/1 -> BitBasher/2
  Real In/1 -> BitBasher/1
  cplx_add6/1(im) -> Gateway Out2/1
  cplx_add6/2(re) -> Gateway Out1/1
  cplx mult1/2(xWi) -> cplx_add/1(a_im)
  cplx mult/2(xWi) -> cplx_add/2(b_im)
  cplx mult1/1(xWr) -> cplx_add/3(a_re)
  cplx mult/1(xWr) -> cplx_add/4(b_re)
  cplx_add/1(im) -> cplx_add1/2(b_im)
  cplx_add/2(re) -> cplx_add1/4(b_re)
  cplx mult2/2(xWi) -> cplx_add1/1(a_im)
  cplx mult2/1(xWr) -> cplx_add1/3(a_re)
  cplx_add1/2(re) -> cplx_add2/4(b_re)
  cplx_add1/1(im) -> cplx_add2/2(b_im)
  cplx mult3/2(xWi) -> cplx_add2/1(a_im)
  cplx mult3/1(xWr) -> cplx_add2/3(a_re)
  cplx_add2/2(re) -> cplx_add3/4(b_re)
  cplx_add2/1(im) -> cplx_add3/2(b_im)
  cplx mult4/1(xWr) -> cplx_add3/3(a_re)
  cplx mult4/2(xWi) -> cplx_add3/1(a_im)
  cplx_add3/2(re) -> cplx_add4/4(b_re)
  cplx_add3/1(im) -> cplx_add4/2(b_im)
  cplx mult5/1(xWr) -> cplx_add4/3(a_re)
  cplx mult5/2(xWi) -> cplx_add4/1(a_im)
  cplx_add4/2(re) -> cplx_add5/4(b_re)
  cplx_add4/1(im) -> cplx_add5/2(b_im)
  cplx mult6/1(xWr) -> cplx_add5/3(a_re)
  cplx mult6/2(xWi) -> cplx_add5/1(a_im)
  cplx_add5/2(re) -> cplx_add6/4(b_re)
  cplx_add5/1(im) -> cplx_add6/2(b_im)
  cplx mult7/2(xWi) -> cplx_add6/1(a_im)
  cplx mult7/1(xWr) -> cplx_add6/3(a_re)
  cplx_add13/1(im) -> Gateway Out4/1
  cplx_add13/2(re) -> Gateway Out3/1
  cplx mult9/2(xWi) -> cplx_add7/1(a_im)
  cplx mult8/2(xWi) -> cplx_add7/2(b_im)
  cplx mult9/1(xWr) -> cplx_add7/3(a_re)
  cplx mult8/1(xWr) -> cplx_add7/4(b_re)
  cplx_add7/1(im) -> cplx_add8/2(b_im)
  cplx_add7/2(re) -> cplx_add8/4(b_re)
  cplx mult10/2(xWi) -> cplx_add8/1(a_im)
  cplx mult10/1(xWr) -> cplx_add8/3(a_re)
  cplx_add8/2(re) -> cplx_add9/4(b_re)
  cplx_add8/1(im) -> cplx_add9/2(b_im)
  cplx mult11/2(xWi) -> cplx_add9/1(a_im)
  cplx mult11/1(xWr) -> cplx_add9/3(a_re)
  cplx_add9/2(re) -> cplx_add10/4(b_re)
  cplx_add9/1(im) -> cplx_add10/2(b_im)
  cplx mult12/1(xWr) -> cplx_add10/3(a_re)
  cplx mult12/2(xWi) -> cplx_add10/1(a_im)
  cplx_add10/2(re) -> cplx_add11/4(b_re)
  cplx_add10/1(im) -> cplx_add11/2(b_im)
  cplx mult13/1(xWr) -> cplx_add11/3(a_re)
  cplx mult13/2(xWi) -> cplx_add11/1(a_im)
  cplx_add11/2(re) -> cplx_add12/4(b_re)
  cplx_add11/1(im) -> cplx_add12/2(b_im)
  cplx mult14/1(xWr) -> cplx_add12/3(a_re)
  cplx mult14/2(xWi) -> cplx_add12/1(a_im)
  cplx_add12/2(re) -> cplx_add13/4(b_re)
  cplx_add12/1(im) -> cplx_add13/2(b_im)
  cplx mult15/2(xWi) -> cplx_add13/1(a_im)
  cplx mult15/1(xWr) -> cplx_add13/3(a_re)
  cplx_add17/1(im) -> Gateway Out6/1
  cplx_add17/2(re) -> Gateway Out5/1
  cplx mult23/2(xWi) -> cplx_add18/1(a_im)
  cplx mult22/2(xWi) -> cplx_add18/2(b_im)
  cplx mult23/1(xWr) -> cplx_add18/3(a_re)
  cplx mult22/1(xWr) -> cplx_add18/4(b_re)
  cplx_add18/1(im) -> cplx_add19/2(b_im)
  cplx_add18/2(re) -> cplx_add19/4(b_re)
  cplx mult16/2(xWi) -> cplx_add19/1(a_im)
  cplx mult16/1(xWr) -> cplx_add19/3(a_re)
  cplx_add19/2(re) -> cplx_add20/4(b_re)
  cplx_add19/1(im) -> cplx_add20/2(b_im)
  cplx mult17/2(xWi) -> cplx_add20/1(a_im)
  cplx mult17/1(xWr) -> cplx_add20/3(a_re)
  cplx_add20/2(re) -> cplx_add14/4(b_re)
  cplx_add20/1(im) -> cplx_add14/2(b_im)
  cplx mult18/1(xWr) -> cplx_add14/3(a_re)
  cplx mult18/2(xWi) -> cplx_add14/1(a_im)
  cplx_add14/2(re) -> cplx_add15/4(b_re)
  cplx_add14/1(im) -> cplx_add15/2(b_im)
  cplx mult19/1(xWr) -> cplx_add15/3(a_re)
  cplx mult19/2(xWi) -> cplx_add15/1(a_im)
  cplx_add15/2(re) -> cplx_add16/4(b_re)
  cplx_add15/1(im) -> cplx_add16/2(b_im)
  cplx mult20/1(xWr) -> cplx_add16/3(a_re)
  cplx mult20/2(xWi) -> cplx_add16/1(a_im)
  cplx_add16/2(re) -> cplx_add17/4(b_re)
  cplx_add16/1(im) -> cplx_add17/2(b_im)
  cplx mult21/2(xWi) -> cplx_add17/1(a_im)
  cplx mult21/1(xWr) -> cplx_add17/3(a_re)
  cplx_add24/1(im) -> Gateway Out8/1
  cplx_add24/2(re) -> Gateway Out7/1
  cplx mult31/2(xWi) -> cplx_add25/1(a_im)
  cplx mult30/2(xWi) -> cplx_add25/2(b_im)
  cplx mult31/1(xWr) -> cplx_add25/3(a_re)
  cplx mult30/1(xWr) -> cplx_add25/4(b_re)
  cplx_add25/1(im) -> cplx_add26/2(b_im)
  cplx_add25/2(re) -> cplx_add26/4(b_re)
  cplx mult24/2(xWi) -> cplx_add26/1(a_im)
  cplx mult24/1(xWr) -> cplx_add26/3(a_re)
  cplx_add26/2(re) -> cplx_add27/4(b_re)
  cplx_add26/1(im) -> cplx_add27/2(b_im)
  cplx mult25/2(xWi) -> cplx_add27/1(a_im)
  cplx mult25/1(xWr) -> cplx_add27/3(a_re)
  cplx_add27/2(re) -> cplx_add21/4(b_re)
  cplx_add27/1(im) -> cplx_add21/2(b_im)
  cplx mult26/1(xWr) -> cplx_add21/3(a_re)
  cplx mult26/2(xWi) -> cplx_add21/1(a_im)
  cplx_add21/2(re) -> cplx_add22/4(b_re)
  cplx_add21/1(im) -> cplx_add22/2(b_im)
  cplx mult27/1(xWr) -> cplx_add22/3(a_re)
  cplx mult27/2(xWi) -> cplx_add22/1(a_im)
  cplx_add22/2(re) -> cplx_add23/4(b_re)
  cplx_add22/1(im) -> cplx_add23/2(b_im)
  cplx mult28/1(xWr) -> cplx_add23/3(a_re)
  cplx mult28/2(xWi) -> cplx_add23/1(a_im)
  cplx_add23/2(re) -> cplx_add24/4(b_re)
  cplx_add23/1(im) -> cplx_add24/2(b_im)
  cplx mult29/2(xWi) -> cplx_add24/1(a_im)
  cplx mult29/1(xWr) -> cplx_add24/3(a_re)
  cplx_add31/1(im) -> Gateway Out10/1
  cplx_add31/2(re) -> Gateway Out9/1
  cplx mult39/2(xWi) -> cplx_add32/1(a_im)
  cplx mult38/2(xWi) -> cplx_add32/2(b_im)
  cplx mult39/1(xWr) -> cplx_add32/3(a_re)
  cplx mult38/1(xWr) -> cplx_add32/4(b_re)
  cplx_add32/1(im) -> cplx_add33/2(b_im)
  cplx_add32/2(re) -> cplx_add33/4(b_re)
  cplx mult32/2(xWi) -> cplx_add33/1(a_im)
  cplx mult32/1(xWr) -> cplx_add33/3(a_re)
  cplx_add33/2(re) -> cplx_add34/4(b_re)
  cplx_add33/1(im) -> cplx_add34/2(b_im)
  cplx mult33/2(xWi) -> cplx_add34/1(a_im)
  cplx mult33/1(xWr) -> cplx_add34/3(a_re)
  cplx_add34/2(re) -> cplx_add28/4(b_re)
  cplx_add34/1(im) -> cplx_add28/2(b_im)
  cplx mult34/1(xWr) -> cplx_add28/3(a_re)
  cplx mult34/2(xWi) -> cplx_add28/1(a_im)
  cplx_add28/2(re) -> cplx_add29/4(b_re)
  cplx_add28/1(im) -> cplx_add29/2(b_im)
  cplx mult35/1(xWr) -> cplx_add29/3(a_re)
  cplx mult35/2(xWi) -> cplx_add29/1(a_im)
  cplx_add29/2(re) -> cplx_add30/4(b_re)
  cplx_add29/1(im) -> cplx_add30/2(b_im)
  cplx mult36/1(xWr) -> cplx_add30/3(a_re)
  cplx mult36/2(xWi) -> cplx_add30/1(a_im)
  cplx_add30/2(re) -> cplx_add31/4(b_re)
  cplx_add30/1(im) -> cplx_add31/2(b_im)
  cplx mult37/2(xWi) -> cplx_add31/1(a_im)
  cplx mult37/1(xWr) -> cplx_add31/3(a_re)
  cplx_add38/1(im) -> Gateway Out12/1
  cplx_add38/2(re) -> Gateway Out11/1
  cplx mult47/2(xWi) -> cplx_add39/1(a_im)
  cplx mult46/2(xWi) -> cplx_add39/2(b_im)
  cplx mult47/1(xWr) -> cplx_add39/3(a_re)
  cplx mult46/1(xWr) -> cplx_add39/4(b_re)
  cplx_add39/1(im) -> cplx_add40/2(b_im)
  cplx_add39/2(re) -> cplx_add40/4(b_re)
  cplx mult40/2(xWi) -> cplx_add40/1(a_im)
  cplx mult40/1(xWr) -> cplx_add40/3(a_re)
  cplx_add40/2(re) -> cplx_add41/4(b_re)
  cplx_add40/1(im) -> cplx_add41/2(b_im)
  cplx mult41/2(xWi) -> cplx_add41/1(a_im)
  cplx mult41/1(xWr) -> cplx_add41/3(a_re)
  cplx_add41/2(re) -> cplx_add35/4(b_re)
  cplx_add41/1(im) -> cplx_add35/2(b_im)
  cplx mult42/1(xWr) -> cplx_add35/3(a_re)
  cplx mult42/2(xWi) -> cplx_add35/1(a_im)
  cplx_add35/2(re) -> cplx_add36/4(b_re)
  cplx_add35/1(im) -> cplx_add36/2(b_im)
  cplx mult43/1(xWr) -> cplx_add36/3(a_re)
  cplx mult43/2(xWi) -> cplx_add36/1(a_im)
  cplx_add36/2(re) -> cplx_add37/4(b_re)
  cplx_add36/1(im) -> cplx_add37/2(b_im)
  cplx mult44/1(xWr) -> cplx_add37/3(a_re)
  cplx mult44/2(xWi) -> cplx_add37/1(a_im)
  cplx_add37/2(re) -> cplx_add38/4(b_re)
  cplx_add37/1(im) -> cplx_add38/2(b_im)
  cplx mult45/2(xWi) -> cplx_add38/1(a_im)
  cplx mult45/1(xWr) -> cplx_add38/3(a_re)
  cplx_add45/1(im) -> Gateway Out14/1
  cplx_add45/2(re) -> Gateway Out13/1
  cplx mult55/2(xWi) -> cplx_add46/1(a_im)
  cplx mult54/2(xWi) -> cplx_add46/2(b_im)
  cplx mult55/1(xWr) -> cplx_add46/3(a_re)
  cplx mult54/1(xWr) -> cplx_add46/4(b_re)
  cplx_add46/1(im) -> cplx_add47/2(b_im)
  cplx_add46/2(re) -> cplx_add47/4(b_re)
  cplx mult48/2(xWi) -> cplx_add47/1(a_im)
  cplx mult48/1(xWr) -> cplx_add47/3(a_re)
  cplx_add47/2(re) -> cplx_add48/4(b_re)
  cplx_add47/1(im) -> cplx_add48/2(b_im)
  cplx mult49/2(xWi) -> cplx_add48/1(a_im)
  cplx mult49/1(xWr) -> cplx_add48/3(a_re)
  cplx_add48/2(re) -> cplx_add42/4(b_re)
  cplx_add48/1(im) -> cplx_add42/2(b_im)
  cplx mult50/1(xWr) -> cplx_add42/3(a_re)
  cplx mult50/2(xWi) -> cplx_add42/1(a_im)
  cplx_add42/2(re) -> cplx_add43/4(b_re)
  cplx_add42/1(im) -> cplx_add43/2(b_im)
  cplx mult51/1(xWr) -> cplx_add43/3(a_re)
  cplx mult51/2(xWi) -> cplx_add43/1(a_im)
  cplx_add43/2(re) -> cplx_add44/4(b_re)
  cplx_add43/1(im) -> cplx_add44/2(b_im)
  cplx mult52/1(xWr) -> cplx_add44/3(a_re)
  cplx mult52/2(xWi) -> cplx_add44/1(a_im)
  cplx_add44/2(re) -> cplx_add45/4(b_re)
  cplx_add44/1(im) -> cplx_add45/2(b_im)
  cplx mult53/2(xWi) -> cplx_add45/1(a_im)
  cplx mult53/1(xWr) -> cplx_add45/3(a_re)
  cplx_add52/1(im) -> Gateway Out16/1
  cplx_add52/2(re) -> Gateway Out15/1
  cplx mult63/2(xWi) -> cplx_add53/1(a_im)
  cplx mult62/2(xWi) -> cplx_add53/2(b_im)
  cplx mult63/1(xWr) -> cplx_add53/3(a_re)
  cplx mult62/1(xWr) -> cplx_add53/4(b_re)
  cplx_add53/1(im) -> cplx_add54/2(b_im)
  cplx_add53/2(re) -> cplx_add54/4(b_re)
  cplx mult56/2(xWi) -> cplx_add54/1(a_im)
  cplx mult56/1(xWr) -> cplx_add54/3(a_re)
  cplx_add54/2(re) -> cplx_add55/4(b_re)
  cplx_add54/1(im) -> cplx_add55/2(b_im)
  cplx mult57/2(xWi) -> cplx_add55/1(a_im)
  cplx mult57/1(xWr) -> cplx_add55/3(a_re)
  cplx_add55/2(re) -> cplx_add49/4(b_re)
  cplx_add55/1(im) -> cplx_add49/2(b_im)
  cplx mult58/1(xWr) -> cplx_add49/3(a_re)
  cplx mult58/2(xWi) -> cplx_add49/1(a_im)
  cplx_add49/2(re) -> cplx_add50/4(b_re)
  cplx_add49/1(im) -> cplx_add50/2(b_im)
  cplx mult59/1(xWr) -> cplx_add50/3(a_re)
  cplx mult59/2(xWi) -> cplx_add50/1(a_im)
  cplx_add50/2(re) -> cplx_add51/4(b_re)
  cplx_add50/1(im) -> cplx_add51/2(b_im)
  cplx mult60/1(xWr) -> cplx_add51/3(a_re)
  cplx mult60/2(xWi) -> cplx_add51/1(a_im)
  cplx_add51/2(re) -> cplx_add52/4(b_re)
  cplx_add51/1(im) -> cplx_add52/2(b_im)
  cplx mult61/2(xWi) -> cplx_add52/1(a_im)
  cplx mult61/1(xWr) -> cplx_add52/3(a_re)
  Delay1/1 -> cplx mult1/1(x), cplx mult9/1(x), cplx mult23/1(x), cplx mult31/1(x), cplx mult39/1(x), cplx mult55/1(x), cplx mult63/1(x), cplx mult47/1(x), Delay7/1, Capture Delay Line Inputs/2(xin_1)
  Delay7/1 -> cplx mult2/1(x), cplx mult10/1(x), cplx mult16/1(x), cplx mult24/1(x), cplx mult40/1(x), cplx mult48/1(x), cplx mult56/1(x), cplx mult32/1(x), Delay2/1, Capture Delay Line Inputs/3(xin_2)
  Gateway Out2/1 -> Capture X0 Outputs/1(In1)
  Gateway Out1/1 -> Capture X0 Outputs/2(In2)
  Gateway Out4/1 -> Capture X1 Outputs/1(In1)
  Gateway Out3/1 -> Capture X1 Outputs/2(In2)
  Sine Wave/1 -> Real In/1
  Constant/1 -> Imaginary In/1
  Gateway Out6/1 -> Capture X2 Outputs/1(In1)
  Gateway Out5/1 -> Capture X2 Outputs/2(In2)
  Gateway Out8/1 -> Capture X3 Outputs/1(In1)
  Gateway Out7/1 -> Capture X3 Outputs/2(In2)
  Gateway Out10/1 -> Capture X4 Outputs/1(In1)
  Gateway Out9/1 -> Capture X4 Outputs/2(In2)
  Gateway Out12/1 -> Capture X5 Outputs/1(In1)
  Gateway Out11/1 -> Capture X5 Outputs/2(In2)
  Gateway Out14/1 -> Capture X6 Outputs/1(In1)
  Gateway Out13/1 -> Capture X6 Outputs/2(In2)
  Gateway Out16/1 -> Capture X7 Outputs/1(In1)
  Gateway Out15/1 -> Capture X7 Outputs/2(In2)
